simulink model "PMSM_Model-2"  (R2021a)
settings: Solver=VariableStepAuto  StartTime=0.0  StopTime=0.15  RelTol=1e-3
undefined symbols (not defined in the file): B, J, Lambda_m, Ld, Lq, P, Rs, Td
libraries: spsPermanentMagnetSynchronousMachineLib x1, spsThreePhaseProgrammableVoltageSourceLib x1, spspowerguiLib x1
settings Model: Creator=ziad allam  LastModifiedBy=ziad allam

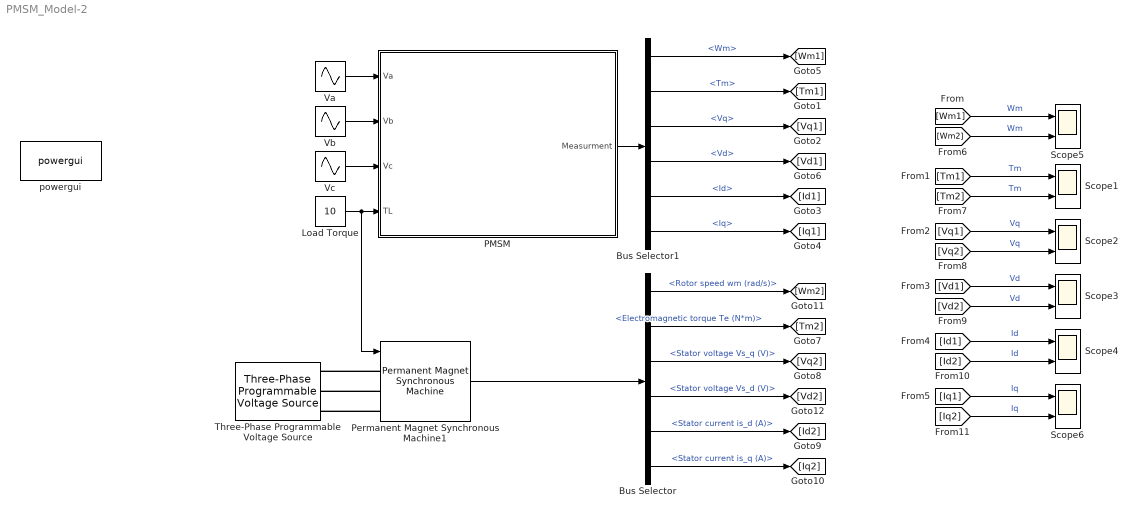
== system PMSM_Model-2 ==
  Bus Selector : BusSelector  OutputSignals=Rotor speed wm (rad/s),Electromagnetic torque Te (N*m),Stator voltage Vs_q (V),Stator voltage Vs_d (V),Stator current is_d (A),Stator current is_q (A)
  Bus Selector1 : BusSelector  OutputSignals=Wm,Tm,Vq,Vd,Id,Iq
  Load Torque : Constant  Value=10
  PMSM : Subsystem
  Permanent Magnet Synchronous Machine1 : spsPermanentMagnetSynchronousMachineLib/Permanent Magnet Synchronous Machine  NbPhases=3  FluxDistribution=Sinusoidal  RotorType=Salient-pole  MechanicalLoad=Torque Tm  PresetModel=No  ShowDetailedParameters=on  MeasurementBus=off  Resistance=Rs  Inductance=8.5e-3  dqInductances=[Ld Lq]  La=(Ld*Lq)/2  MachineConstant=Flux linkage established by magnets (V.s)  Flux=Lambda_m  VoltageCst=44.6195  TorqueCst=0.369  Flat=120  Mechanical=[J B 2 0]  PolePairs=4  InitialConditions=[0,0, 0,0]  InitialConditions5ph=[0 0 0 0 0 0]  RefAngle=90 degrees behind phase A axis (modified Park)  IterativeDiscreteModel=Trapezoidal non iterative  TsBlock=-1  TsPowergui=0
  Scope{1..6} (6 alike) : Scope  NumInputPorts=2
  Three-Phase Programmable Voltage Source : spsThreePhaseProgrammableVoltageSourceLib/Three-Phase Programmable Voltage Source  PositiveSequence="[220  0 50]"  VariationEntity=None  VariationType=Table of time-amplitude pairs  VariationTypeAlt=Step  VariationStep=0.5  VariationRate=10  VariationMagnitude=0.3  VariationFrequency=2  VariationTiming=[1 2]  VariationPhaseA=off  Amplitudes=[1 0.8 1.2 1.0]  TimeValues=[0 0.1 0.15 0.2]  HarmonicGeneration=off  HarmonicA=[3 0.2 -25 0]  HarmonicB=[2 0.15 35 2]  Timing="[0.05  3]"  BusType=swing  Pref=0  Qref=0  Qmin=-inf  Qmax=inf
  Va : Sin  Amplitude=220  Frequency=2*pi*50  SampleTime=0
  Vb : Sin  Amplitude=220  Frequency=2*pi*50  Phase=-2*pi/3  SampleTime=0
  Vc : Sin  Amplitude=220  Frequency=2*pi*50  Phase=2*pi/3  SampleTime=0
  powergui : spspowerguiLib/powergui  Priority=1  SimulationMode=Continuous  SampleTime=50e-6  frequency=60  Iterations=50  frequencyindice=50  Pbase=100e6  ErrMax=1e-4  UnitsV=kV  UnitsW=MW  buscounter=0  FunctionMessages=off  echomessages=off  EnableUseOfTLC=off  CurrentSourceSwitches=off  DisableSnubberDevices=off  DisableRonSwitches=off  DisableVfSwitches=off  DisplayEquations=off  AutomaticDiscreteSolvers=off  SolverType=Tustin/Backward Euler (TBE)  Interpol=off  ExternalGateDelay=off  methode=off  Ts=100  x0status=blocks  SPID=on  SwTol=0  HookPort=off  NonlinearTolerance=1e-4  nMaxIteration=100  ContinueOnMaxIteration=off  RestoreLinks=warning  ResistiveCurrentMeasurement=off  Frange=[0:2:500]  Ylog=off  Xlog=on  ShowGrid=off  save=off  variable=ZData  structure=0  ZoomFFT=off  StartTime=0.0  cycles=1  DisplayStyle=1  fundamental=60  FreqAxis=off  MaxFrequency=1000  frequencyindicesteady=1  RmsSteady=1  display=off
  wires:
  Load Torque/1 -> PMSM/4(TL), Permanent Magnet Synchronous Machine1/1
  Permanent Magnet Synchronous Machine1/1 -> Bus Selector/1
  Va/1 -> PMSM/1(Va)
  Vb/1 -> PMSM/2(Vb)
  Vc/1 -> PMSM/3(Vc)
  PMSM/1(Measurment) -> Bus Selector1/1
  [Iq1] -> Scope6/1  "Iq"
  [Id1] -> Scope4/1  "Id"
  [Vq1] -> Scope2/1  "Vq"
  [Vd1] -> Scope3/1  "Vd"
  [Wm1] -> Scope5/1  "Wm"
  [Tm1] -> Scope1/1  "Tm"
  Bus Selector1/1 -> [Wm1]  "<Wm>"
  Bus Selector/1 -> [Wm2]  "<Rotor speed wm (rad/s)>"
  Bus Selector/2 -> [Tm2]  "<Electromagnetic torque Te (N*m)>"
  Bus Selector/3 -> [Vq2]  "<Stator voltage Vs_q (V)>"
  Bus Selector/4 -> [Vd2]  "<Stator voltage Vs_d (V)>"
  Bus Selector/5 -> [Id2]  "<Stator current is_d (A)>"
  Bus Selector/6 -> [Iq2]  "<Stator current is_q (A)>"
  Bus Selector1/2 -> [Tm1]  "<Tm>"
  Bus Selector1/3 -> [Vq1]  "<Vq>"
  Bus Selector1/4 -> [Vd1]  "<Vd>"
  Bus Selector1/6 -> [Iq1]  "<Iq>"
  Bus Selector1/5 -> [Id1]  "<Id>"
  [Vq2] -> Scope2/2  "Vq"
  [Vd2] -> Scope3/2  "Vd"
  [Id2] -> Scope4/2  "Id"
  [Iq2] -> Scope6/2  "Iq"
  [Tm2] -> Scope1/2  "Tm"
  [Wm2] -> Scope5/2  "Wm"
  connections:
  Permanent Magnet Synchronous Machine1/LConn1 -- Three-Phase Programmable Voltage Source/RConn1
  Permanent Magnet Synchronous Machine1/LConn2 -- Three-Phase Programmable Voltage Source/RConn2
  Permanent Magnet Synchronous Machine1/LConn3 -- Three-Phase Programmable Voltage Source/RConn3

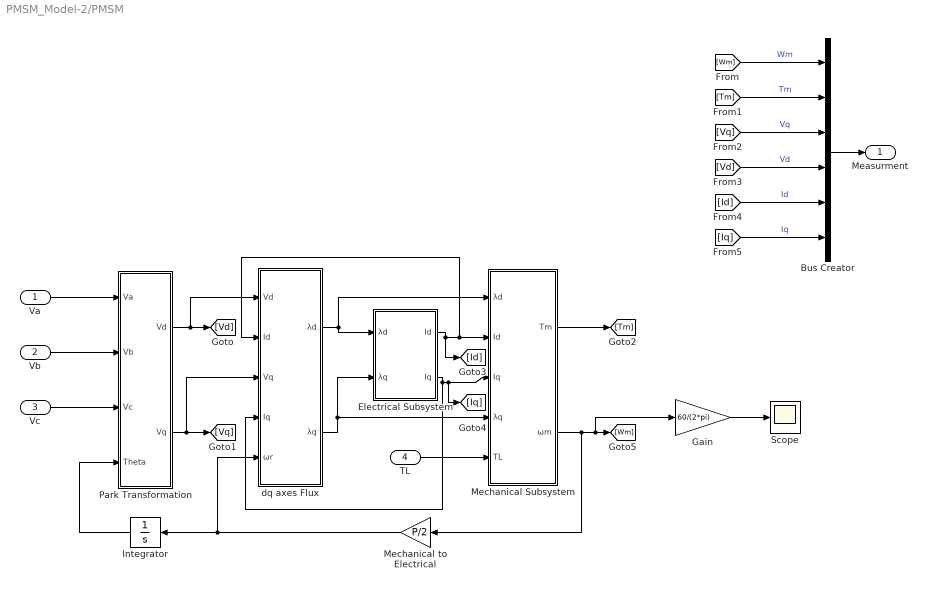
== system PMSM_Model-2/PMSM ==
  Va : Inport
  Vb : Inport  Port=2
  Vc : Inport  Port=3
  TL : Inport  Port=4
  Bus Creator : BusCreator  Inputs=6
  Electrical Subsystem : Subsystem
  Gain : Gain  Gain=60/(2*pi)
  Integrator : Integrator
  Mechanical Subsystem : Subsystem
  "Mechanical to Electrical " : Gain  Gain=P/2
  Park Transformation : Subsystem
  Scope : Scope
  dq axes Flux : Subsystem
  Measurment : Outport
  wires:
  Vb/1 -> Park Transformation/2(Vb)
  Mechanical Subsystem/2(ωm) -> Gain/1, [Wm], "Mechanical to Electrical "/1
  Electrical Subsystem/1(Id) -> dq axes Flux/2(Id), Mechanical Subsystem/2(Id), [Id]
  "Mechanical to Electrical "/1 -> dq axes Flux/5(ωr), Integrator/1
  dq axes Flux/1(λd) -> Mechanical Subsystem/1(λd), Electrical Subsystem/1(λd)
  Va/1 -> Park Transformation/1(Va)
  Mechanical Subsystem/1(Tm) -> [Tm]
  dq axes Flux/2(λq) -> Electrical Subsystem/2(λq), Mechanical Subsystem/4(λq)
  Vc/1 -> Park Transformation/3(Vc)
  Electrical Subsystem/2(Iq) -> [Iq], Mechanical Subsystem/3(Iq), dq axes Flux/4(Iq)
  Integrator/1 -> Park Transformation/4(Theta)
  TL/1 -> Mechanical Subsystem/5(TL)
  [Vq] -> Bus Creator/3  "Vq"
  [Iq] -> Bus Creator/6  "Iq"
  [Wm] -> Bus Creator/1  "Wm"
  [Tm] -> Bus Creator/2  "Tm"
  [Vd] -> Bus Creator/4  "Vd"
  [Id] -> Bus Creator/5  "Id"
  Bus Creator/1 -> Measurment/1
  Gain/1 -> Scope/1
  Park Transformation/1(Vd) -> [Vd], dq axes Flux/1(Vd)
  Park Transformation/2(Vq) -> dq axes Flux/3(Vq), [Vq]

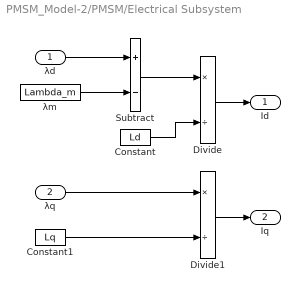
== system PMSM_Model-2/PMSM/Electrical Subsystem ==
  λd : Inport
  λq : Inport  Port=2
  Constant : Constant  Value=Ld
  Constant1 : Constant  Value=Lq
  Divide : Product  Inputs=*/
  Divide1 : Product  Inputs=*/
  Subtract : Sum  Inputs=+-
  λm : Constant  Value=Lambda_m
  Id : Outport
  Iq : Outport  Port=2
  wires:
  λd/1 -> Subtract/1
  λm/1 -> Subtract/2
  Subtract/1 -> Divide/1
  Constant/1 -> Divide/2
  Divide/1 -> Id/1
  λq/1 -> Divide1/1
  Constant1/1 -> Divide1/2
  Divide1/1 -> Iq/1

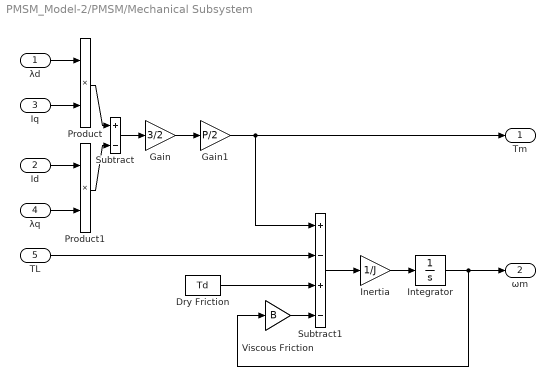
== system PMSM_Model-2/PMSM/Mechanical Subsystem ==
  λd : Inport
  Id : Inport  Port=2
  Iq : Inport  Port=3
  λq : Inport  Port=4
  TL : Inport  Port=5
  Dry Friction : Constant  Value=Td
  Gain : Gain  Gain=3/2
  Gain1 : Gain  Gain=P/2
  Inertia : Gain  Gain=1/J
  Integrator : Integrator
  Product : Product
  Product1 : Product
  Subtract : Sum  Inputs=+-
  Subtract1 : Sum  Inputs=+-+-
  Viscous Friction : Gain  Gain=B
  Tm : Outport
  ωm : Outport  Port=2
  wires:
  λd/1 -> Product/1
  λq/1 -> Product1/2
  Product/1 -> Subtract/1
  Product1/1 -> Subtract/2
  Subtract/1 -> Gain/1
  Gain/1 -> Gain1/1
  Gain1/1 -> Subtract1/1, Tm/1
  TL/1 -> Subtract1/2
  Viscous Friction/1 -> Subtract1/4
  Subtract1/1 -> Inertia/1
  Inertia/1 -> Integrator/1
  Integrator/1 -> ωm/1, Viscous Friction/1
  Dry Friction/1 -> Subtract1/3
  Iq/1 -> Product/2
  Id/1 -> Product1/1

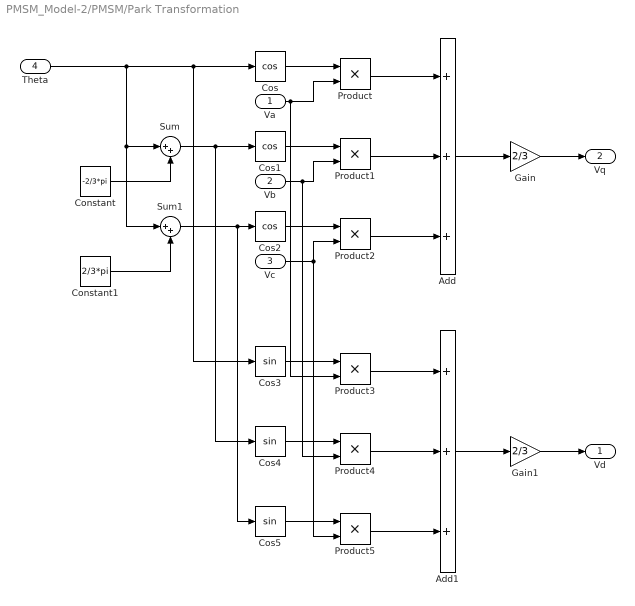
== system PMSM_Model-2/PMSM/Park Transformation ==
  Va : Inport
  Vb : Inport  Port=2
  Vc : Inport  Port=3
  Theta : Inport  Port=4
  Add : Sum  Inputs=+++
  Add1 : Sum  Inputs=+++
  Constant : Constant  Value=-2/3*pi
  Constant1 : Constant  Value=2/3*pi
  Cos : Trigonometry  Operator=cos
  Cos1 : Trigonometry  Operator=cos
  Cos2 : Trigonometry  Operator=cos
  Cos3 : Trigonometry
  Cos4 : Trigonometry
  Cos5 : Trigonometry
  Gain : Gain  Gain=2/3
  Gain1 : Gain  Gain=2/3
  Product{,1..5} (6 alike) : Product
  Sum : Sum  Inputs=|++
  Sum1 : Sum  Inputs=|++
  Vd : Outport
  Vq : Outport  Port=2
  wires:
  Cos/1 -> Product/1
  Cos1/1 -> Product1/1
  Cos2/1 -> Product2/1
  Constant/1 -> Sum/2
  Constant1/1 -> Sum1/2
  Product1/1 -> Add/2
  Product/1 -> Add/1
  Product2/1 -> Add/3
  Product4/1 -> Add1/2
  Product5/1 -> Add1/3
  Sum/1 -> Cos1/1, Cos4/1
  Vb/1 -> Product4/2, Product1/2
  Theta/1 -> Sum/1, Sum1/1, Cos/1, Cos3/1
  Vc/1 -> Product5/2, Product2/2
  Product3/1 -> Add1/1
  Cos3/1 -> Product3/1
  Va/1 -> Product3/2, Product/2
  Cos4/1 -> Product4/1
  Cos5/1 -> Product5/1
  Sum1/1 -> Cos5/1, Cos2/1
  Add/1 -> Gain/1
  Add1/1 -> Gain1/1
  Gain/1 -> Vq/1
  Gain1/1 -> Vd/1

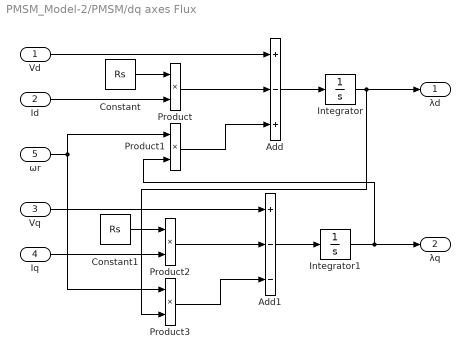
== system PMSM_Model-2/PMSM/dq axes Flux ==
  Vd : Inport
  Id : Inport  Port=2
  Vq : Inport  Port=3
  Iq : Inport  Port=4
  ωr : Inport  Port=5
  Add : Sum  Inputs=+-+
  Add1 : Sum  Inputs=+--
  Constant : Constant  Value=Rs
  Constant1 : Constant  Value=Rs
  Integrator : Integrator
  Integrator1 : Integrator
  Product{,1..3} (4 alike) : Product
  λd : Outport
  λq : Outport  Port=2
  wires:
  Vd/1 -> Add/1
  Constant/1 -> Product/1
  Id/1 -> Product/2
  Product/1 -> Add/2
  Product1/1 -> Add/3
  Add/1 -> Integrator/1
  Integrator/1 -> λd/1, Product3/2
  Product2/1 -> Add1/2
  Vq/1 -> Add1/1
  Product3/1 -> Add1/3
  ωr/1 -> Product3/1, Product1/1
  Constant1/1 -> Product2/1
  Iq/1 -> Product2/2
  Add1/1 -> Integrator1/1
  Integrator1/1 -> λq/1, Product1/2
